simulink model "building_PHPP_carnot83"  (R2023b)
settings: Solver=ode23s  StartTime=-building.preruntime+8760*3600  StopTime=building.runtime+8760*3600  EnableMultiTasking=on
StartFcn:
  | tic
StopFcn:
  | toc
values from neighbouring files (symbols this model uses):
  building = obj    [BUILDING.m]    (also in create_building_automatic.m = building.save(); ini_building_automatic.m = building.add_variant_hvac(building.variant_hvac, hvac); load_building_automatic.m = building.save())
  cp = str2num(value)    [CONSTRUCTION.m]
  p = [timevec_weather weather(:,12)]    [BOUNDARY.m]    (also in WEATHER.m = 0; init_carnotUIBK.m = cell2mat(carnotUIBKpaths(i,2)))
  rho = str2num(value)    [CONSTRUCTION.m]    (also in theta_ground_v1.m = 2000)
undefined symbols (not defined in the file or in its folder): Dreifach, get_building, Qdot_C, Qdot_C_energy, Qdot_H, Qdot_H_energy, Qdot_I_electricity, Qdot_I_electricity_energy, Qdot_I_light, Qdot_I_light_energy, Qdot_I_person, Qdot_I_person_energy, Qdot_S, Qdot_S_energy, Qdot_T_ground, Qdot_T_ground_energy, Qdot_T_neighbour, Qdot_T_neighbour_energy, Qdot_T_opaque, Qdot_T_opaque_energy, Qdot_T_window, Qdot_T_window_energy, Qdot_V_infiltration, Qdot_V_infiltration_energy, Qdot_V_mech, Qdot_V_mech_energy, Qdot_V_window, Qdot_V_window_energy, Tc, Tr, Ts, Wärmeschutzglas, x_CO2, x_H2O, x_VOC
libraries: carnotUIBK x2418, carnot x1
(part 1 of 32)
settings Model: SimulationMode=accelerator  Creator=c8461199  LastModifiedBy=c8461246
settings SolverCC: AlgebraicLoopSolver=TrustRegion
settings DataIOCC: SaveOutput=off  SignalLogging=off  DSMLogging=off  VisualizeSimOutput=off  SaveTime=off  ReturnWorkspaceOutputs=off
settings OptimizationCC: LifeSpan=inf  SimCompilerOptimization=on
settings DebuggingCC: MaxConsecutiveZCsMsg=warning  UnconnectedInputMsg=warning  UnconnectedOutputMsg=warning  UnconnectedLineMsg=warning  AllowSymbolicDim=off  SFUnexpectedBacktrackingDiag=warning  SFNoUnconditionalDefaultTransitionDiag=warning  SFExecutionAtInitializationDiag=none  ArithmeticOperatorsInVariantConditions=warning
settings ModelReferenceCC: EnableRefExpFcnMdlSchedulingChecks=on  EnableParallelModelReferenceBuilds=on  ParallelModelReferenceMATLABWorkerInit=Copy Base Workspace  PropagateSignalLabelsOutOfModel=off
settings SFSimCC: SimUserSources=carlib.c  SimUseLocalCustomCode=off  CustomCodeUndefinedFunction=UseInterfaceOnly
settings RTWCC: RTWUseLocalCustomCode=off  BuildConfiguration=Faster Runs
settings CodeAppCC: StateflowObjectComments=on
settings GRTTargetCC: TargetLangStandard=C89/C90 (ANSI)
settings ConfigComp: CovMetricSettings=dw  CovSaveCumulativeToWorkspaceVar=on  CovSaveSingleToWorkspaceVar=on  CovExternalEMLEnable=off

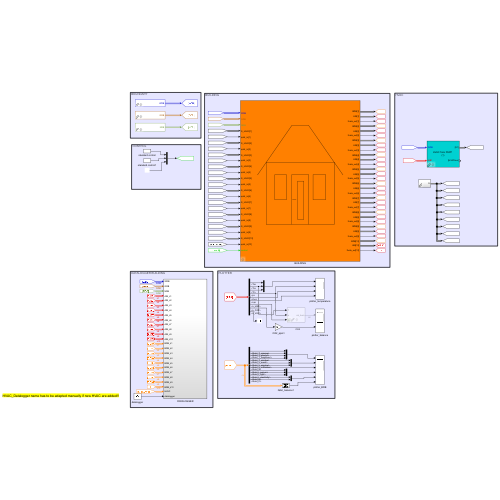
[thumbnail: Simulink's stored preview of the top-level diagram]
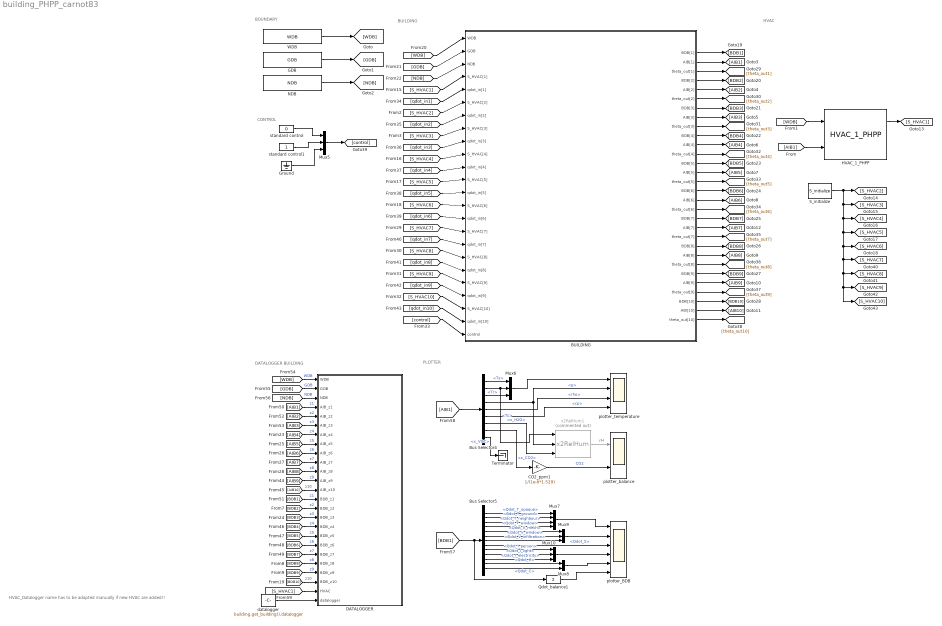
== system building_PHPP_carnot83 ==
  note: HVAC_Datalogger name has to be adapted manually if new HVAC are added!!
  note: PLOTTER
  note: CONTROL
  note: DATALOGGER BUILDING
  note: HVAC
  note: BUILDING
  note: BOUNDARY
  BUILDING : Subsystem  mask{building=get_building(building)}
      mask prompts: building "BUILDING object"
      mask init:
      | b = building;
      mask Display:
      | plot(-20,-30,120,100,[10,10,90,90,10],[0,50,50,0,0],...
      |     [100,60,40,0],[40,80,80,40],[20,34,34,20,20],[40,40,20,20,40],...
      |     [60,60,40,40],[0,40,40,0],[65,80,80,65,65],[40,40,20,20,40],...
      |     [47,54,54,47,47],[35,35,4,4,35],[45,41],[20,20])
  Bus Selector4 : BusSelector  OutputSignals=Ts,Tc,Tr,p,rho,cp,x_H2O,x_CO2,x_VOC
  Bus Selector5 : BusSelector  OutputSignals=Qdot_T_opaque,Qdot_T_ground,Qdot_T_neighbour,Qdot_T_window,Qdot_V_mech,Qdot_V_window,Qdot_V_infiltration,Qdot_S,Qdot_I_person,Qdot_I_light,Qdot_I_electricity,Qdot_H,Qdot_C
  CO2_ppm1 : Gain  Gain=1/(1e-6*1.529)
  DATALOGGER : Subsystem
  GDB : carnotUIBK/boundary/GDB  building=get_building(building)
  Ground : Ground
  HVAC_1_PHPP : carnotUIBK/HVAC/HVAC_1_PHPP  building=get_building(building)  system=1
  Mux10 : Mux  Inputs=3
  Mux5 : Mux  Inputs=[1 1 18]
  Mux6 : Mux  Inputs=3
  Mux7 : Mux
  Mux8 : Mux  Inputs=2
  Mux9 : Mux  Inputs=3
  NDB : carnotUIBK/boundary/NDB  building=get_building(building)
  Qdot_balance1 : Sum  Inputs=1
  S_initialize : carnotUIBK/general/S_initialize  SystemSampleTime=-1  VariantActivationTime=update diagram  AllowFlexibleInterface=on  Latency=0  AutoFrameSizeCalculation=off
  Terminator : Terminator
  WDB : carnotUIBK/boundary/WDB  building=get_building(building)
  datalogger : Constant  Value=building.get_building().datalogger
  plotter_BDB : Scope  NumInputPorts=6
  plotter_balance : Scope  NumInputPorts=2
  plotter_temperature : Scope  NumInputPorts=4
  standard control : Constant  Value=0
  standard control1 : Constant
  x2RelHum1 : carnot/Basic/Material_Properties/x2RelHum  Commented=on
      settings: SourceProductName=Carnot
  wires:
  WDB/1 -> [WDB]
  GDB/1 -> [GDB]
  NDB/1 -> [NDB]
  [WDB] -> BUILDING/1(WDB)
  [GDB] -> BUILDING/2(GDB)
  [NDB] -> BUILDING/3(NDB)
  BUILDING/2(AIB[1]) -> [AIB1]
  BUILDING/5(AIB[2]) -> [AIB2]
  BUILDING/8(AIB[3]) -> [AIB3]
  BUILDING/11(AIB[4]) -> [AIB4]
  BUILDING/14(AIB[5]) -> [AIB5]
  BUILDING/17(AIB[6]) -> [AIB6]
  BUILDING/29(AIB[10]) -> [AIB10]
  BUILDING/26(AIB[9]) -> [AIB9]
  BUILDING/23(AIB[8]) -> [AIB8]
  BUILDING/20(AIB[7]) -> [AIB7]
  [S_HVAC5] -> BUILDING/12(S_HVAC[5])
  [S_HVAC4] -> BUILDING/10(S_HVAC[4])
  [AIB1] -> HVAC_1_PHPP/2
  [S_HVAC1] -> BUILDING/4(S_HVAC[1])
  [S_HVAC2] -> BUILDING/6(S_HVAC[2])
  [S_HVAC3] -> BUILDING/8(S_HVAC[3])
  [S_HVAC6] -> BUILDING/14(S_HVAC[6])
  HVAC_1_PHPP/1 -> [S_HVAC1]
  [S_HVAC10] -> BUILDING/22(S_HVAC[10])
  [S_HVAC9] -> BUILDING/20(S_HVAC[9])
  [S_HVAC8] -> BUILDING/18(S_HVAC[8])
  [S_HVAC7] -> BUILDING/16(S_HVAC[7])
  [control] -> BUILDING/24(control)
  BUILDING/1(BDB[1]) -> [BDB1]
  BUILDING/28(BDB[10]) -> [BDB10]
  BUILDING/4(BDB[2]) -> [BDB2]
  BUILDING/7(BDB[3]) -> [BDB3]
  BUILDING/10(BDB[4]) -> [BDB4]
  BUILDING/13(BDB[5]) -> [BDB5]
  BUILDING/16(BDB[6]) -> [BDB6]
  BUILDING/19(BDB[7]) -> [BDB7]
  BUILDING/22(BDB[8]) -> [BDB8]
  BUILDING/25(BDB[9]) -> [BDB9]
  [qdot_in1] -> BUILDING/5(qdot_in[1])
  [qdot_in9] -> BUILDING/21(qdot_in[9])
  [qdot_in10] -> BUILDING/23(qdot_in[10])
  [qdot_in8] -> BUILDING/19(qdot_in[8])
  [qdot_in7] -> BUILDING/17(qdot_in[7])
  [qdot_in6] -> BUILDING/15(qdot_in[6])
  [qdot_in4] -> BUILDING/11(qdot_in[4])
  [qdot_in5] -> BUILDING/13(qdot_in[5])
  [qdot_in3] -> BUILDING/9(qdot_in[3])
  [qdot_in2] -> BUILDING/7(qdot_in[2])
  BUILDING/3(theta_out[1]) -> [theta_out1]
  BUILDING/30(theta_out[10]) -> [theta_out10]
  BUILDING/27(theta_out[9]) -> [theta_out9]
  BUILDING/24(theta_out[8]) -> [theta_out8]
  BUILDING/21(theta_out[7]) -> [theta_out7]
  BUILDING/18(theta_out[6]) -> [theta_out6]
  BUILDING/15(theta_out[5]) -> [theta_out5]
  BUILDING/12(theta_out[4]) -> [theta_out4]
  BUILDING/9(theta_out[3]) -> [theta_out3]
  BUILDING/6(theta_out[2]) -> [theta_out2]
  datalogger/1 -> DATALOGGER/25(datalogger)
  standard control/1 -> Mux5/1
  Mux5/1 -> [control]
  Ground/1 -> Mux5/3
  [AIB1] -> DATALOGGER/4(AIB_z1)  "z1"
  [WDB] -> DATALOGGER/1(WDB)  "WDB"
  [GDB] -> DATALOGGER/2(GDB)  "GDB"
  [NDB] -> DATALOGGER/3(NDB)  "NDB"
  [AIB2] -> DATALOGGER/5(AIB_z2)  "z2"
  [AIB3] -> DATALOGGER/6(AIB_z3)  "z3"
  [AIB4] -> DATALOGGER/7(AIB_z4)  "z4"
  [AIB5] -> DATALOGGER/8(AIB_z5)  "z5"
  [AIB6] -> DATALOGGER/9(AIB_z6)  "z6"
  [AIB7] -> DATALOGGER/10(AIB_z7)  "z7"
  [AIB8] -> DATALOGGER/11(AIB_z8)  "z8"
  [AIB9] -> DATALOGGER/12(AIB_z9)  "z9"
  [AIB10] -> DATALOGGER/13(AIB_z10)  "z10"
  [BDB1] -> DATALOGGER/14(BDB_z1)  "z1"
  [BDB2] -> DATALOGGER/15(BDB_z2)  "z2"
  [BDB3] -> DATALOGGER/16(BDB_z3)  "z3"
  [BDB4] -> DATALOGGER/17(BDB_z4)  "z4"
  [BDB5] -> DATALOGGER/18(BDB_z5)  "z5"
  [BDB6] -> DATALOGGER/19(BDB_z6)  "z6"
  [BDB7] -> DATALOGGER/20(BDB_z7)  "z7"
  [BDB8] -> DATALOGGER/21(BDB_z8)  "z8"
  [BDB9] -> DATALOGGER/22(BDB_z9)  "z9"
  [BDB10] -> DATALOGGER/23(BDB_z10)  "z10"
  Bus Selector4/4 -> x2RelHum1/2, plotter_temperature/2  "<p>"
  Bus Selector4/1 -> Mux6/1  "<Ts>"
  Bus Selector4/2 -> x2RelHum1/1, Mux6/2  "<Tc>"
  Bus Selector4/3 -> Mux6/3  "<Tr>"
  Mux6/1 -> plotter_temperature/1
  Bus Selector4/5 -> plotter_temperature/3  "<rho>"
  Bus Selector4/6 -> plotter_temperature/4  "<cp>"
  Bus Selector4/8 -> CO2_ppm1/1  "<x_CO2>"
  CO2_ppm1/1 -> plotter_balance/2  "CO2"
  Bus Selector4/7 -> x2RelHum1/3  "<x_H2O>"
  x2RelHum1/1 -> plotter_balance/1  "rH"
  Bus Selector5/6 -> Mux9/2  "<Qdot_V_window>"
  Bus Selector5/5 -> Mux9/1  "<Qdot_V_mech>"
  Bus Selector5/4 -> Mux7/4  "<Qdot_T_window>"
  Bus Selector5/3 -> Mux7/3  "<Qdot_T_neighbour>"
  Bus Selector5/2 -> Mux7/2  "<Qdot_T_ground>"
  Bus Selector5/1 -> Mux7/1  "<Qdot_T_opaque>"
  Bus Selector5/7 -> Mux9/3  "<Qdot_V_infiltration>"
  Bus Selector5/8 -> plotter_BDB/3  "<Qdot_S>"
  Bus Selector5/9 -> Mux10/1  "<Qdot_I_person>"
  Bus Selector5/10 -> Mux10/2  "<Qdot_I_light>"
  Bus Selector5/11 -> Mux10/3  "<Qdot_I_electricity>"
  Mux7/1 -> plotter_BDB/1
  [BDB1] -> Qdot_balance1/1, Bus Selector5/1
  Mux9/1 -> plotter_BDB/2
  Mux10/1 -> plotter_BDB/4
  Bus Selector5/12 -> Mux8/1  "<Qdot_H>"
  Bus Selector5/13 -> Mux8/2  "<Qdot_C>"
  Mux8/1 -> plotter_BDB/5
  Qdot_balance1/1 -> plotter_BDB/6
  [AIB1] -> Bus Selector4/1
  [S_HVAC1] -> DATALOGGER/24(HVAC)
  standard control1/1 -> Mux5/2
  [WDB] -> HVAC_1_PHPP/1
  Bus Selector4/9 -> Terminator/1  "<x_VOC>"
  S_initialize/1 -> [S_HVAC2], [S_HVAC3], [S_HVAC4], [S_HVAC6], [S_HVAC7], [S_HVAC8], [S_HVAC9], [S_HVAC10], [S_HVAC5]

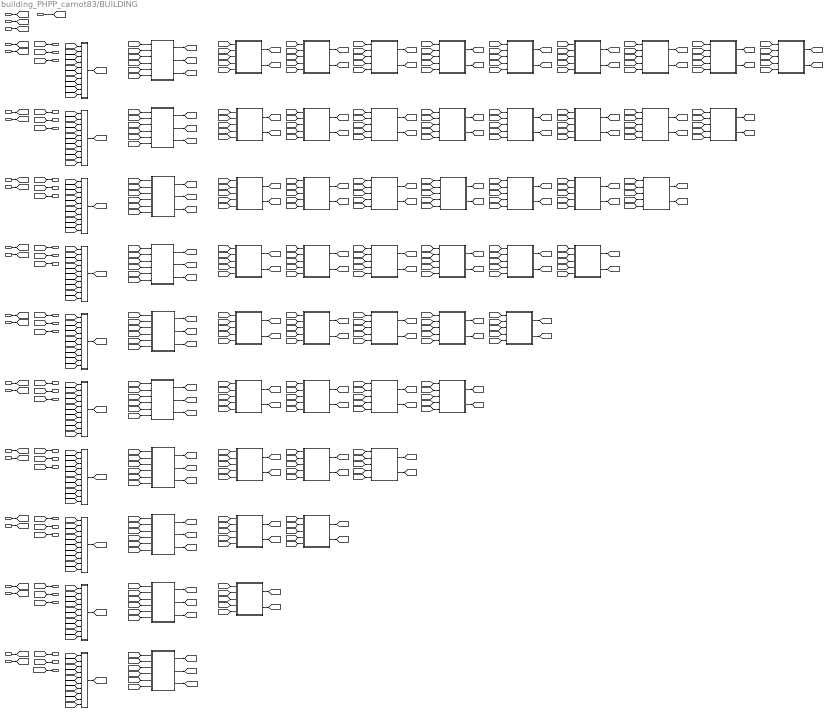
== system building_PHPP_carnot83/BUILDING ==
  note: INTERSECTION 1_2
  note: ZONE 1
  note: ZONE 1 - SUM UP S
  note: ZONE 6 - INPUT AND OUTPUT
  note: ZONE 5 - INPUT AND OUTPUT
  note: ZONE 4 - INPUT AND OUTPUT
  note: ZONE 3 - INPUT AND OUTPUT
  note: ZONE 2 - INPUT AND OUTPUT
  note: ZONE 1 - INPUT AND OUTPUT
  note: BUS BOUNDARY
  note: ZONE 2 - SUM UP S
  note: ZONE 3 - SUM UP S
  note: ZONE 4 - SUM UP S
  note: ZONE 5 - SUM UP S
  note: ZONE 6 - SUM UP S
  note: ZONE 7 - INPUT AND OUTPUT
  note: ZONE 7 - SUM UP S
  note: ZONE 8 - INPUT AND OUTPUT
  note: ZONE 8 - SUM UP S
  note: ZONE 9 - INPUT AND OUTPUT
  note: ZONE 9 - SUM UP S
  note: ZONE 10 - INPUT AND OUTPUT
  note: ZONE 10 - SUM UP S
  note: ZONE 2
  note: ZONE 3
  note: ZONE 4
  note: ZONE 5
  note: ZONE6
  note: ZONE 7
  note: ZONE 8
  note: ZONE 9
  note: ZONE 10
  note: CONTROL
  note: INTERSECTION 1_10
  note: INTERSECTION 1_3
  note: INTERSECTION 1_4
  note: INTERSECTION 1_5
  note: INTERSECTION 1_6
  note: INTERSECTION 1_7
  note: INTERSECTION 1_8
  note: INTERSECTION 1_9
  note: INTERSECTION 2_3
  note: INTERSECTION 2_9
  note: INTERSECTION 2_10
  note: INTERSECTION 2_4
  note: INTERSECTION 2_5
  note: INTERSECTION 2_6
  note: INTERSECTION 2_7
  note: INTERSECTION 2_8
  note: INTERSECTION 3_4
  note: INTERSECTION 3_5
  note: INTERSECTION 3_6
  note: INTERSECTION 3_7
  note: INTERSECTION 3_8
  note: INTERSECTION 3_9
  note: INTERSECTION 3_10
  note: INTERSECTION 4_5
  note: INTERSECTION 4_6
  note: INTERSECTION 4_7
  note: INTERSECTION 4_8
  note: INTERSECTION 4_9
  note: INTERSECTION 4_10
  note: INTERSECTION 5_6
  note: INTERSECTION 5_7
  note: INTERSECTION 5_8
  note: INTERSECTION 5_9
  note: INTERSECTION 5_10
  note: INTERSECTION 6_7
  note: INTERSECTION 6_8
  note: INTERSECTION 6_9
  note: INTERSECTION 6_10
  note: INTERSECTION 7_8
  note: INTERSECTION 7_9
  note: INTERSECTION 7_10
  note: INTERSECTION 8_9
  note: INTERSECTION 8_10
  note: INTERSECTION 9_10
  WDB : Inport
  GDB : Inport  Port=2
  NDB : Inport  Port=3
  S_HVAC[1] : Inport  Port=4
  qdot_in[1] : Inport  Port=5
  S_HVAC[2] : Inport  Port=6
  qdot_in[2] : Inport  Port=7
  S_HVAC[3] : Inport  Port=8
  qdot_in[3] : Inport  Port=9
  S_HVAC[4] : Inport  Port=10
  qdot_in[4] : Inport  Port=11
  S_HVAC[5] : Inport  Port=12
  qdot_in[5] : Inport  Port=13
  S_HVAC[6] : Inport  Port=14
  qdot_in[6] : Inport  Port=15
  S_HVAC[7] : Inport  Port=16
  qdot_in[7] : Inport  Port=17
  S_HVAC[8] : Inport  Port=18
  qdot_in[8] : Inport  Port=19
  S_HVAC[9] : Inport  Port=20
  qdot_in[9] : Inport  Port=21
  S_HVAC[10] : Inport  Port=22
  qdot_in[10] : Inport  Port=23
  control : Inport  Port=24
  INTERSECTION_1_10 : Subsystem  VariantControl=Variant1  mask{intersection=b.thermalzone.intersection{1,10}}
      mask prompts: intersection "INTERSECTION object"
      mask init:
      | i = intersection;
      | z = intersection;
      mask Display: fprintf('%s',intersection.name)
  INTERSECTION_1_2 : Subsystem  VariantControl=Variant1  mask{intersection=b.thermalzone.intersection{1,2}}
      mask prompts: intersection "INTERSECTION object"
      mask init:
      | i = intersection;
      | z = intersection;
      mask Display: fprintf('%s',intersection.name)
  INTERSECTION_1_3 : Subsystem  VariantControl=Variant1  mask{intersection=b.thermalzone.intersection{1,3}}
      mask prompts: intersection "INTERSECTION object"
      mask init:
      | i = intersection;
      | z = intersection;
      mask Display: fprintf('%s',intersection.name)
  INTERSECTION_1_4 : Subsystem  VariantControl=Variant1  mask{intersection=b.thermalzone.intersection{1,4}}
      mask prompts: intersection "INTERSECTION object"
      mask init:
      | i = intersection;
      | z = intersection;
      mask Display: fprintf('%s',intersection.name)
  INTERSECTION_1_5 : Subsystem  VariantControl=Variant1  mask{intersection=b.thermalzone.intersection{1,5}}
      mask prompts: intersection "INTERSECTION object"
      mask init:
      | i = intersection;
      | z = intersection;
      mask Display: fprintf('%s',intersection.name)
  INTERSECTION_1_6 : Subsystem  VariantControl=Variant1  mask{intersection=b.thermalzone.intersection{1,6}}
      mask prompts: intersection "INTERSECTION object"
      mask init:
      | i = intersection;
      | z = intersection;
      mask Display: fprintf('%s',intersection.name)
  INTERSECTION_1_7 : Subsystem  VariantControl=Variant1  mask{intersection=b.thermalzone.intersection{1,7}}
      mask prompts: intersection "INTERSECTION object"
      mask init:
      | i = intersection;
      | z = intersection;
      mask Display: fprintf('%s',intersection.name)
  INTERSECTION_1_8 : Subsystem  VariantControl=Variant1  mask{intersection=b.thermalzone.intersection{1,8}}
      mask prompts: intersection "INTERSECTION object"
      mask init:
      | i = intersection;
      | z = intersection;
      mask Display: fprintf('%s',intersection.name)
  INTERSECTION_1_9 : Subsystem  VariantControl=Variant1  mask{intersection=b.thermalzone.intersection{1,9}}
      mask prompts: intersection "INTERSECTION object"
      mask init:
      | i = intersection;
      | z = intersection;
      mask Display: fprintf('%s',intersection.name)
  INTERSECTION_2_10 : Subsystem  VariantControl=Variant1  mask{intersection=b.thermalzone.intersection{2,10}}
      mask prompts: intersection "INTERSECTION object"
      mask init:
      | i = intersection;
      | z = intersection;
      mask Display: fprintf('%s',intersection.name)
  INTERSECTION_2_3 : Subsystem  VariantControl=Variant1  mask{intersection=b.thermalzone.intersection{2,3}}
      mask prompts: intersection "INTERSECTION object"
      mask init:
      | i = intersection;
      | z = intersection;
      mask Display: fprintf('%s',intersection.name)
  INTERSECTION_2_4 : Subsystem  VariantControl=Variant1  mask{intersection=b.thermalzone.intersection{2,4}}
      mask prompts: intersection "INTERSECTION object"
      mask init:
      | i = intersection;
      | z = intersection;
      mask Display: fprintf('%s',intersection.name)
  INTERSECTION_2_5 : Subsystem  VariantControl=Variant1  mask{intersection=b.thermalzone.intersection{2,5}}
      mask prompts: intersection "INTERSECTION object"
      mask init:
      | i = intersection;
      | z = intersection;
      mask Display: fprintf('%s',intersection.name)
  INTERSECTION_2_6 : Subsystem  VariantControl=Variant1  mask{intersection=b.thermalzone.intersection{2,6}}
      mask prompts: intersection "INTERSECTION object"
      mask init:
      | i = intersection;
      | z = intersection;
      mask Display: fprintf('%s',intersection.name)
  INTERSECTION_2_7 : Subsystem  VariantControl=Variant1  mask{intersection=b.thermalzone.intersection{2,7}}
      mask prompts: intersection "INTERSECTION object"
      mask init:
      | i = intersection;
      | z = intersection;
      mask Display: fprintf('%s',intersection.name)
  INTERSECTION_2_8 : Subsystem  VariantControl=Variant1  mask{intersection=b.thermalzone.intersection{2,8}}
      mask prompts: intersection "INTERSECTION object"
      mask init:
      | i = intersection;
      | z = intersection;
      mask Display: fprintf('%s',intersection.name)
  INTERSECTION_2_9 : Subsystem  VariantControl=Variant1  mask{intersection=b.thermalzone.intersection{2,9}}
      mask prompts: intersection "INTERSECTION object"
      mask init:
      | i = intersection;
      | z = intersection;
      mask Display: fprintf('%s',intersection.name)
  INTERSECTION_3_10 : Subsystem  VariantControl=Variant1  mask{intersection=b.thermalzone.intersection{3,10}}
      mask prompts: intersection "INTERSECTION object"
      mask init:
      | i = intersection;
      | z = intersection;
      mask Display: fprintf('%s',intersection.name)
  INTERSECTION_3_4 : Subsystem  VariantControl=Variant1  mask{intersection=b.thermalzone.intersection{3,4}}
      mask prompts: intersection "INTERSECTION object"
      mask init:
      | i = intersection;
      | z = intersection;
      mask Display: fprintf('%s',intersection.name)
  INTERSECTION_3_5 : Subsystem  VariantControl=Variant1  mask{intersection=b.thermalzone.intersection{3,5}}
      mask prompts: intersection "INTERSECTION object"
      mask init:
      | i = intersection;
      | z = intersection;
      mask Display: fprintf('%s',intersection.name)
  INTERSECTION_3_6 : Subsystem  VariantControl=Variant1  mask{intersection=b.thermalzone.intersection{3,6}}
      mask prompts: intersection "INTERSECTION object"
      mask init:
      | i = intersection;
      | z = intersection;
      mask Display: fprintf('%s',intersection.name)
  INTERSECTION_3_7 : Subsystem  VariantControl=Variant1  mask{intersection=b.thermalzone.intersection{3,7}}
      mask prompts: intersection "INTERSECTION object"
      mask init:
      | i = intersection;
      | z = intersection;
      mask Display: fprintf('%s',intersection.name)
  INTERSECTION_3_8 : Subsystem  VariantControl=Variant1  mask{intersection=b.thermalzone.intersection{3,8}}
      mask prompts: intersection "INTERSECTION object"
      mask init:
      | i = intersection;
      | z = intersection;
      mask Display: fprintf('%s',intersection.name)
  INTERSECTION_3_9 : Subsystem  VariantControl=Variant1  mask{intersection=b.thermalzone.intersection{3,9}}
      mask prompts: intersection "INTERSECTION object"
      mask init:
      | i = intersection;
      | z = intersection;
      mask Display: fprintf('%s',intersection.name)
  INTERSECTION_4_10 : Subsystem  VariantControl=Variant1  mask{intersection=b.thermalzone.intersection{4,10}}
      mask prompts: intersection "INTERSECTION object"
      mask init:
      | i = intersection;
      | z = intersection;
      mask Display: fprintf('%s',intersection.name)
  INTERSECTION_4_5 : Subsystem  VariantControl=Variant1  mask{intersection=b.thermalzone.intersection{4,5}}
      mask prompts: intersection "INTERSECTION object"
      mask init:
      | i = intersection;
      | z = intersection;
      mask Display: fprintf('%s',intersection.name)
  INTERSECTION_4_6 : Subsystem  VariantControl=Variant1  mask{intersection=b.thermalzone.intersection{4,6}}
      mask prompts: intersection "INTERSECTION object"
      mask init:
      | i = intersection;
      | z = intersection;
      mask Display: fprintf('%s',intersection.name)
  INTERSECTION_4_7 : Subsystem  VariantControl=Variant1  mask{intersection=b.thermalzone.intersection{4,7}}
      mask prompts: intersection "INTERSECTION object"
      mask init:
      | i = intersection;
      | z = intersection;
      mask Display: fprintf('%s',intersection.name)
  INTERSECTION_4_8 : Subsystem  VariantControl=Variant1  mask{intersection=b.thermalzone.intersection{4,8}}
      mask prompts: intersection "INTERSECTION object"
      mask init:
      | i = intersection;
      | z = intersection;
      mask Display: fprintf('%s',intersection.name)
  INTERSECTION_4_9 : Subsystem  VariantControl=Variant1  mask{intersection=b.thermalzone.intersection{4,9}}
      mask prompts: intersection "INTERSECTION object"
      mask init:
      | i = intersection;
      | z = intersection;
      mask Display: fprintf('%s',intersection.name)
  INTERSECTION_5_10 : Subsystem  VariantControl=Variant1  mask{intersection=b.thermalzone.intersection{5,10}}
      mask prompts: intersection "INTERSECTION object"
      mask init:
      | i = intersection;
      | z = intersection;
      mask Display: fprintf('%s',intersection.name)
  INTERSECTION_5_6 : Subsystem  VariantControl=Variant1  mask{intersection=b.thermalzone.intersection{5,6}}
      mask prompts: intersection "INTERSECTION object"
      mask init:
      | i = intersection;
      | z = intersection;
      mask Display: fprintf('%s',intersection.name)
  INTERSECTION_5_7 : Subsystem  VariantControl=Variant1  mask{intersection=b.thermalzone.intersection{5,7}}
      mask prompts: intersection "INTERSECTION object"
      mask init:
      | i = intersection;
      | z = intersection;
      mask Display: fprintf('%s',intersection.name)
  INTERSECTION_5_8 : Subsystem  VariantControl=Variant1  mask{intersection=b.thermalzone.intersection{5,8}}
      mask prompts: intersection "INTERSECTION object"
      mask init:
      | i = intersection;
      | z = intersection;
      mask Display: fprintf('%s',intersection.name)
  INTERSECTION_5_9 : Subsystem  VariantControl=Variant1  mask{intersection=b.thermalzone.intersection{5,9}}
      mask prompts: intersection "INTERSECTION object"
      mask init:
      | i = intersection;
      | z = intersection;
      mask Display: fprintf('%s',intersection.name)
  INTERSECTION_6_10 : Subsystem  VariantControl=Variant1  mask{intersection=b.thermalzone.intersection{6,10}}
      mask prompts: intersection "INTERSECTION object"
      mask init:
      | i = intersection;
      | z = intersection;
      mask Display: fprintf('%s',intersection.name)
  INTERSECTION_6_7 : Subsystem  VariantControl=Variant1  mask{intersection=b.thermalzone.intersection{6,7}}
      mask prompts: intersection "INTERSECTION object"
      mask init:
      | i = intersection;
      | z = intersection;
      mask Display: fprintf('%s',intersection.name)
  INTERSECTION_6_8 : Subsystem  VariantControl=Variant1  mask{intersection=b.thermalzone.intersection{6,8}}
      mask prompts: intersection "INTERSECTION object"
      mask init:
      | i = intersection;
      | z = intersection;
      mask Display: fprintf('%s',intersection.name)
  INTERSECTION_6_9 : Subsystem  VariantControl=Variant1  mask{intersection=b.thermalzone.intersection{6,9}}
      mask prompts: intersection "INTERSECTION object"
      mask init:
      | i = intersection;
      | z = intersection;
      mask Display: fprintf('%s',intersection.name)
  INTERSECTION_7_10 : Subsystem  VariantControl=Variant1  mask{intersection=b.thermalzone.intersection{7,10}}
      mask prompts: intersection "INTERSECTION object"
      mask init:
      | i = intersection;
      | z = intersection;
      mask Display: fprintf('%s',intersection.name)
  INTERSECTION_7_8 : Subsystem  VariantControl=Variant1  mask{intersection=b.thermalzone.intersection{7,8}}
      mask prompts: intersection "INTERSECTION object"
      mask init:
      | i = intersection;
      | z = intersection;
      mask Display: fprintf('%s',intersection.name)
  INTERSECTION_7_9 : Subsystem  VariantControl=Variant1  mask{intersection=b.thermalzone.intersection{7,9}}
      mask prompts: intersection "INTERSECTION object"
      mask init:
      | i = intersection;
      | z = intersection;
      mask Display: fprintf('%s',intersection.name)
  INTERSECTION_8_10 : Subsystem  VariantControl=Variant1  mask{intersection=b.thermalzone.intersection{8,10}}
      mask prompts: intersection "INTERSECTION object"
      mask init:
      | i = intersection;
      | z = intersection;
      mask Display: fprintf('%s',intersection.name)
  INTERSECTION_8_9 : Subsystem  VariantControl=Variant1  mask{intersection=b.thermalzone.intersection{8,9}}
      mask prompts: intersection "INTERSECTION object"
      mask init:
      | i = intersection;
      | z = intersection;
      mask Display: fprintf('%s',intersection.name)
  INTERSECTION_9_10 : Subsystem  VariantControl=Variant1  mask{intersection=b.thermalzone.intersection{9,10}}
      mask prompts: intersection "INTERSECTION object"
      mask init:
      | i = intersection;
      | z = intersection;
      mask Display: fprintf('%s',intersection.name)
  Subsystem : Subsystem
  Subsystem1 : Subsystem
  Subsystem2 : Subsystem
  Subsystem3 : Subsystem
  Subsystem4 : Subsystem
  Subsystem5 : Subsystem
  Subsystem6 : Subsystem
  Subsystem7 : Subsystem
  Subsystem8 : Subsystem
  Subsystem9 : Subsystem
  ZONE_1 : Subsystem  mask{zone=b.thermalzone.zone(1)}
      mask prompts: zone "ZONE object"
      mask init:
      | z = zone;
      mask Display: fprintf('%s',zone.name)
  ZONE_10 : Subsystem  mask{zone=b.thermalzone.zone(10)}
      mask prompts: zone "ZONE object"
      mask init:
      | z = zone;
      mask Display: fprintf('%s',zone.name)
  ZONE_2 : Subsystem  mask{zone=b.thermalzone.zone(2)}
      mask prompts: zone "ZONE object"
      mask init:
      | z = zone;
      mask Display: fprintf('%s',zone.name)
  ZONE_3 : Subsystem  mask{zone=b.thermalzone.zone(3)}
      mask prompts: zone "ZONE object"
      mask init:
      | z = zone;
      mask Display: fprintf('%s',zone.name)
  ZONE_4 : Subsystem  mask{zone=b.thermalzone.zone(4)}
      mask prompts: zone "ZONE object"
      mask init:
      | z = zone;
      mask Display: fprintf('%s',zone.name)
  ZONE_5 : Subsystem  mask{zone=b.thermalzone.zone(5)}
      mask prompts: zone "ZONE object"
      mask init:
      | z = zone;
      mask Display: fprintf('%s',zone.name)
  ZONE_6 : Subsystem  mask{zone=b.thermalzone.zone(6)}
      mask prompts: zone "ZONE object"
      mask init:
      | z = zone;
      mask Display: fprintf('%s',zone.name)
  ZONE_7 : Subsystem  mask{zone=b.thermalzone.zone(7)}
      mask prompts: zone "ZONE object"
      mask init:
      | z = zone;
      mask Display: fprintf('%s',zone.name)
  ZONE_8 : Subsystem  mask{zone=b.thermalzone.zone(8)}
      mask prompts: zone "ZONE object"
      mask init:
      | z = zone;
      mask Display: fprintf('%s',zone.name)
  ZONE_9 : Subsystem  mask{zone=b.thermalzone.zone(9)}
      mask prompts: zone "ZONE object"
      mask init:
      | z = zone;
      mask Display: fprintf('%s',zone.name)
  BDB[1] : Outport  VectorParamsAs1DForOutWhenUnconnected=off
  AIB[1] : Outport  Port=2  VectorParamsAs1DForOutWhenUnconnected=off
  theta_out[1] : Outport  Port=3  VectorParamsAs1DForOutWhenUnconnected=off
  BDB[2] : Outport  Port=4  VectorParamsAs1DForOutWhenUnconnected=off
  AIB[2] : Outport  Port=5  VectorParamsAs1DForOutWhenUnconnected=off
  theta_out[2] : Outport  Port=6  VectorParamsAs1DForOutWhenUnconnected=off
  BDB[3] : Outport  Port=7  VectorParamsAs1DForOutWhenUnconnected=off
  AIB[3] : Outport  Port=8  VectorParamsAs1DForOutWhenUnconnected=off
  theta_out[3] : Outport  Port=9  VectorParamsAs1DForOutWhenUnconnected=off
  BDB[4] : Outport  Port=10  VectorParamsAs1DForOutWhenUnconnected=off
  AIB[4] : Outport  Port=11  VectorParamsAs1DForOutWhenUnconnected=off
  theta_out[4] : Outport  Port=12  VectorParamsAs1DForOutWhenUnconnected=off
  BDB[5] : Outport  Port=13  VectorParamsAs1DForOutWhenUnconnected=off
  AIB[5] : Outport  Port=14  VectorParamsAs1DForOutWhenUnconnected=off
  theta_out[5] : Outport  Port=15  VectorParamsAs1DForOutWhenUnconnected=off
  BDB[6] : Outport  Port=16  VectorParamsAs1DForOutWhenUnconnected=off
  AIB[6] : Outport  Port=17  VectorParamsAs1DForOutWhenUnconnected=off
  theta_out[6] : Outport  Port=18  VectorParamsAs1DForOutWhenUnconnected=off
  BDB[7] : Outport  Port=19  VectorParamsAs1DForOutWhenUnconnected=off
  AIB[7] : Outport  Port=20  VectorParamsAs1DForOutWhenUnconnected=off
  theta_out[7] : Outport  Port=21  VectorParamsAs1DForOutWhenUnconnected=off
  BDB[8] : Outport  Port=22  VectorParamsAs1DForOutWhenUnconnected=off
  AIB[8] : Outport  Port=23  VectorParamsAs1DForOutWhenUnconnected=off
  theta_out[8] : Outport  Port=24  VectorParamsAs1DForOutWhenUnconnected=off
  BDB[9] : Outport  Port=25  VectorParamsAs1DForOutWhenUnconnected=off
  AIB[9] : Outport  Port=26  VectorParamsAs1DForOutWhenUnconnected=off
  theta_out[9] : Outport  Port=27  VectorParamsAs1DForOutWhenUnconnected=off
  BDB[10] : Outport  Port=28  VectorParamsAs1DForOutWhenUnconnected=off
  AIB[10] : Outport  Port=29  VectorParamsAs1DForOutWhenUnconnected=off
  theta_out[10] : Outport  Port=30  VectorParamsAs1DForOutWhenUnconnected=off
  wires:
  WDB/1 -> [WDB]
  GDB/1 -> [GDB]
  NDB/1 -> [NDB]
  S_HVAC[1]/1 -> [S_HVAC_1]
  qdot_in[1]/1 -> [qdot_in_1]
  [BDB_1] -> BDB[1]/1
  [AIB_1] -> AIB[1]/1
  [theta_out_1z] -> theta_out[1]/1
  S_HVAC[2]/1 -> [S_HVAC_2]
  qdot_in[2]/1 -> [qdot_in_2]
  qdot_in[3]/1 -> [qdot_in_3]
  S_HVAC[3]/1 -> [S_HVAC_3]
  S_HVAC[4]/1 -> [S_HVAC_4]
  qdot_in[4]/1 -> [qdot_in_4]
  S_HVAC[5]/1 -> [S_HVAC_5]
  qdot_in[5]/1 -> [qdot_in_5]
  qdot_in[6]/1 -> [qdot_in_6]
  S_HVAC[6]/1 -> [S_HVAC_6]
  [BDB_2] -> BDB[2]/1
  [AIB_2] -> AIB[2]/1
  [theta_out_2z] -> theta_out[2]/1
  [BDB_3] -> BDB[3]/1
  [AIB_3] -> AIB[3]/1
  [theta_out_3z] -> theta_out[3]/1
  [BDB_4] -> BDB[4]/1
  [AIB_4] -> AIB[4]/1
  [theta_out_4z] -> theta_out[4]/1
  [BDB_5] -> BDB[5]/1
  [AIB_5] -> AIB[5]/1
  [theta_out_5z] -> theta_out[5]/1
  [BDB_6] -> BDB[6]/1
  [AIB_6] -> AIB[6]/1
  [theta_out_6z] -> theta_out[6]/1
  ZONE_1/1(BDB) -> [BDB_1]
  ZONE_1/2(AIB) -> [AIB_1]
  ZONE_1/3(theta_out) -> [theta_out_1z]
  [qdot_in_1] -> ZONE_1/5(Qdot_in)
  [S_in_1] -> ZONE_1/4(S_in)
  [GDB] -> ZONE_1/2(GDB)
  [NDB] -> ZONE_1/3(NDB)
  [S_HVAC_1] -> Subsystem/1(S1)
  [S_I_16] -> Subsystem/6(S6)
  [S_I_12] -> Subsystem/2(S2)
  [S_I_13] -> Subsystem/3(S3)
  [S_I_14] -> Subsystem/4(S4)
  [S_I_15] -> Subsystem/5(S5)
  Subsystem/1(Sout) -> [S_in_1]
  [S_HVAC_2] -> Subsystem1/1(S1)
  Subsystem1/1(Sout) -> [S_in_2]
  Subsystem2/1(Sout) -> [S_in_3]
  Subsystem3/1(Sout) -> [S_in_4]
  Subsystem4/1(Sout) -> [S_in_5]
  Subsystem5/1(Sout) -> [S_in_6]
  [S_I_17] -> Subsystem/7(S7)
  [S_I_18] -> Subsystem/8(S8)
  [S_I_19] -> Subsystem/9(S9)
  [S_I_110] -> Subsystem/10(S10)
  [S_I_27] -> Subsystem1/7(S7)
  [S_I_28] -> Subsystem1/8(S8)
  [S_I_29] -> Subsystem1/9(S9)
  [S_I_210] -> Subsystem1/10(S10)
  [S_I_21] -> Subsystem1/2(S2)
  [S_I_23] -> Subsystem1/3(S3)
  [S_I_26] -> Subsystem1/6(S6)
  [S_I_25] -> Subsystem1/5(S5)
  [S_I_24] -> Subsystem1/4(S4)
  [S_I_37] -> Subsystem2/7(S7)
  [S_I_38] -> Subsystem2/8(S8)
  [S_I_39] -> Subsystem2/9(S9)
  [S_I_310] -> Subsystem2/10(S10)
  [S_HVAC_3] -> Subsystem2/1(S1)
  [S_I_31] -> Subsystem2/2(S2)
  [S_I_32] -> Subsystem2/3(S3)
  [S_I_34] -> Subsystem2/4(S4)
  [S_I_35] -> Subsystem2/5(S5)
  [S_I_36] -> Subsystem2/6(S6)
  [S_I_47] -> Subsystem3/7(S7)
  [S_I_48] -> Subsystem3/8(S8)
  [S_I_49] -> Subsystem3/9(S9)
  [S_I_410] -> Subsystem3/10(S10)
  [S_HVAC_4] -> Subsystem3/1(S1)
  [S_I_41] -> Subsystem3/2(S2)
  [S_I_42] -> Subsystem3/3(S3)
  [S_I_43] -> Subsystem3/4(S4)
  [S_I_45] -> Subsystem3/5(S5)
  [S_I_46] -> Subsystem3/6(S6)
  [S_I_57] -> Subsystem4/7(S7)
  [S_I_58] -> Subsystem4/8(S8)
  [S_I_59] -> Subsystem4/9(S9)
  [S_I_510] -> Subsystem4/10(S10)
  [S_HVAC_5] -> Subsystem4/1(S1)
  [S_I_51] -> Subsystem4/2(S2)
  [S_I_52] -> Subsystem4/3(S3)
  [S_I_53] -> Subsystem4/4(S4)
  [S_I_54] -> Subsystem4/5(S5)
  [S_I_56] -> Subsystem4/6(S6)
  [S_I_67] -> Subsystem5/7(S7)
  [S_I_68] -> Subsystem5/8(S8)
  [S_I_69] -> Subsystem5/9(S9)
  [S_I_610] -> Subsystem5/10(S10)
  [S_HVAC_6] -> Subsystem5/1(S1)
  [S_I_61] -> Subsystem5/2(S2)
  [S_I_62] -> Subsystem5/3(S3)
  [S_I_63] -> Subsystem5/4(S4)
  [S_I_64] -> Subsystem5/5(S5)
  [S_I_65] -> Subsystem5/6(S6)
  qdot_in[7]/1 -> [qdot_in_7]
  S_HVAC[7]/1 -> [S_HVAC_7]
  [BDB_7] -> BDB[7]/1
  [AIB_7] -> AIB[7]/1
  [theta_out_7z] -> theta_out[7]/1
  Subsystem6/1(Sout) -> [S_in_7]
  [S_I_76] -> Subsystem6/7(S7)
  [S_I_78] -> Subsystem6/8(S8)
  [S_I_79] -> Subsystem6/9(S9)
  [S_I_710] -> Subsystem6/10(S10)
  [S_HVAC_7] -> Subsystem6/1(S1)
  [S_I_71] -> Subsystem6/2(S2)
  [S_I_72] -> Subsystem6/3(S3)
  [S_I_73] -> Subsystem6/4(S4)
  [S_I_74] -> Subsystem6/5(S5)
  [S_I_75] -> Subsystem6/6(S6)
  qdot_in[8]/1 -> [qdot_in_8]
  S_HVAC[8]/1 -> [S_HVAC_8]
  [BDB_8] -> BDB[8]/1
  [AIB_8] -> AIB[8]/1
  [theta_out_8z] -> theta_out[8]/1
  Subsystem7/1(Sout) -> [S_in_8]
  [S_I_86] -> Subsystem7/7(S7)
  [S_I_87] -> Subsystem7/8(S8)
  [S_I_89] -> Subsystem7/9(S9)
  [S_I_810] -> Subsystem7/10(S10)
  [S_HVAC_8] -> Subsystem7/1(S1)
  [S_I_81] -> Subsystem7/2(S2)
  [S_I_82] -> Subsystem7/3(S3)
  [S_I_83] -> Subsystem7/4(S4)
  [S_I_84] -> Subsystem7/5(S5)
  [S_I_85] -> Subsystem7/6(S6)
  qdot_in[9]/1 -> [qdot_in_9]
  S_HVAC[9]/1 -> [S_HVAC_9]
  [BDB_9] -> BDB[9]/1
  [AIB_9] -> AIB[9]/1
  [theta_out_9z] -> theta_out[9]/1
  Subsystem8/1(Sout) -> [S_in_9]
  [S_I_96] -> Subsystem8/7(S7)
  [S_I_97] -> Subsystem8/8(S8)
  [S_I_98] -> Subsystem8/9(S9)
  [S_I_910] -> Subsystem8/10(S10)
  [S_HVAC_9] -> Subsystem8/1(S1)
  [S_I_91] -> Subsystem8/2(S2)
  [S_I_92] -> Subsystem8/3(S3)
  [S_I_93] -> Subsystem8/4(S4)
  [S_I_94] -> Subsystem8/5(S5)
  [S_I_95] -> Subsystem8/6(S6)
  qdot_in[10]/1 -> [qdot_in_10]
  S_HVAC[10]/1 -> [S_HVAC_10]
  [BDB_10] -> BDB[10]/1
  [AIB_10] -> AIB[10]/1
  [theta_out_10z] -> theta_out[10]/1
  Subsystem9/1(Sout) -> [S_in_10]
  [S_I_106] -> Subsystem9/7(S7)
  [S_I_107] -> Subsystem9/8(S8)
  [S_I_108] -> Subsystem9/9(S9)
  [S_I_109] -> Subsystem9/10(S10)
  [S_HVAC_10] -> Subsystem9/1(S1)
  [S_I_101] -> Subsystem9/2(S2)
  [S_I_102] -> Subsystem9/3(S3)
  [S_I_103] -> Subsystem9/4(S4)
  [S_I_104] -> Subsystem9/5(S5)
  [S_I_105] -> Subsystem9/6(S6)
  ZONE_2/1(BDB) -> [BDB_2]
  ZONE_2/2(AIB) -> [AIB_2]
  ZONE_2/3(theta_out) -> [theta_out_2z]
  [qdot_in_2] -> ZONE_2/5(Qdot_in)
  [S_in_2] -> ZONE_2/4(S_in)
  [GDB] -> ZONE_2/2(GDB)
  [WDB] -> ZONE_2/1(WDB)
  [NDB] -> ZONE_2/3(NDB)
  ZONE_3/1(BDB) -> [BDB_3]
  ZONE_3/2(AIB) -> [AIB_3]
  ZONE_3/3(theta_out) -> [theta_out_3z]
  [qdot_in_3] -> ZONE_3/5(Qdot_in)
  [S_in_3] -> ZONE_3/4(S_in)
  [GDB] -> ZONE_3/2(GDB)
  [WDB] -> ZONE_3/1(WDB)
  [NDB] -> ZONE_3/3(NDB)
  ZONE_4/1(BDB) -> [BDB_4]
  ZONE_4/2(AIB) -> [AIB_4]
  ZONE_4/3(theta_out) -> [theta_out_4z]
  [qdot_in_4] -> ZONE_4/5(Qdot_in)
  [S_in_4] -> ZONE_4/4(S_in)
  [GDB] -> ZONE_4/2(GDB)
  [WDB] -> ZONE_4/1(WDB)
  [NDB] -> ZONE_4/3(NDB)
  ZONE_5/1(BDB) -> [BDB_5]
  ZONE_5/2(AIB) -> [AIB_5]
  ZONE_5/3(theta_out) -> [theta_out_5z]
  [qdot_in_5] -> ZONE_5/5(Qdot_in)
  [S_in_5] -> ZONE_5/4(S_in)
  [GDB] -> ZONE_5/2(GDB)
  [WDB] -> ZONE_5/1(WDB)
  [NDB] -> ZONE_5/3(NDB)
  ZONE_6/1(BDB) -> [BDB_6]
  ZONE_6/2(AIB) -> [AIB_6]
  ZONE_6/3(theta_out) -> [theta_out_6z]
  [qdot_in_6] -> ZONE_6/5(Qdot_in)
  [S_in_6] -> ZONE_6/4(S_in)
  [GDB] -> ZONE_6/2(GDB)
  [WDB] -> ZONE_6/1(WDB)
  [NDB] -> ZONE_6/3(NDB)
  ZONE_7/1(BDB) -> [BDB_7]
  ZONE_7/2(AIB) -> [AIB_7]
  ZONE_7/3(theta_out) -> [theta_out_7z]
  [qdot_in_7] -> ZONE_7/5(Qdot_in)
  [S_in_7] -> ZONE_7/4(S_in)
  [GDB] -> ZONE_7/2(GDB)
  [WDB] -> ZONE_7/1(WDB)
  [NDB] -> ZONE_7/3(NDB)
  ZONE_8/1(BDB) -> [BDB_8]
  ZONE_8/2(AIB) -> [AIB_8]
  ZONE_8/3(theta_out) -> [theta_out_8z]
  [qdot_in_8] -> ZONE_8/5(Qdot_in)
  [S_in_8] -> ZONE_8/4(S_in)
  [GDB] -> ZONE_8/2(GDB)
  [WDB] -> ZONE_8/1(WDB)
  [NDB] -> ZONE_8/3(NDB)
  ZONE_9/1(BDB) -> [BDB_9]
  ZONE_9/2(AIB) -> [AIB_9]
  ZONE_9/3(theta_out) -> [theta_out_9z]
  [qdot_in_9] -> ZONE_9/5(Qdot_in)
  [S_in_9] -> ZONE_9/4(S_in)
  [GDB] -> ZONE_9/2(GDB)
  [WDB] -> ZONE_9/1(WDB)
  [NDB] -> ZONE_9/3(NDB)
  ZONE_10/1(BDB) -> [BDB_10]
  ZONE_10/2(AIB) -> [AIB_10]
  ZONE_10/3(theta_out) -> [theta_out_10z]
  [qdot_in_10] -> ZONE_10/5(Qdot_in)
  [S_in_10] -> ZONE_10/4(S_in)
  [GDB] -> ZONE_10/2(GDB)
  [WDB] -> ZONE_10/1(WDB)
  [NDB] -> ZONE_10/3(NDB)
  [control] -> ZONE_1/6(control)
  control/1 -> [control]
  [AIB_1] -> INTERSECTION_1_2/1(AIB1)
  [AIB_2] -> INTERSECTION_1_2/2(AIB2)
  INTERSECTION_1_2/1(S1) -> [S_I_12]
  INTERSECTION_1_2/2(S2) -> [S_I_21]
  [control] -> ZONE_2/6(control)
  [control] -> ZONE_3/6(control)
  [control] -> ZONE_4/6(control)
  [control] -> ZONE_5/6(control)
  [control] -> ZONE_6/6(control)
  [control] -> ZONE_7/6(control)
  [control] -> ZONE_8/6(control)
  [control] -> ZONE_9/6(control)
  [control] -> ZONE_10/6(control)
  [BDB_1] -> INTERSECTION_1_2/3(BDB1)
  [BDB_2] -> INTERSECTION_1_2/4(BDB2)
  [WDB] -> ZONE_1/1(WDB)
  [control] -> INTERSECTION_1_2/5(control)
  [AIB_1] -> INTERSECTION_1_10/1(AIB1)
  [AIB_10] -> INTERSECTION_1_10/2(AIB2)
  INTERSECTION_1_10/1(S1) -> [S_I_110]
  INTERSECTION_1_10/2(S2) -> [S_I_101]
  [BDB_1] -> INTERSECTION_1_10/3(BDB1)
  [BDB_10] -> INTERSECTION_1_10/4(BDB2)
  [control] -> INTERSECTION_1_10/5(control)
  [AIB_1] -> INTERSECTION_1_3/1(AIB1)
  [AIB_3] -> INTERSECTION_1_3/2(AIB2)
  INTERSECTION_1_3/1(S1) -> [S_I_13]
  INTERSECTION_1_3/2(S2) -> [S_I_31]
  [BDB_1] -> INTERSECTION_1_3/3(BDB1)
  [BDB_3] -> INTERSECTION_1_3/4(BDB2)
  [control] -> INTERSECTION_1_3/5(control)
  [AIB_1] -> INTERSECTION_1_4/1(AIB1)
  [AIB_4] -> INTERSECTION_1_4/2(AIB2)
  INTERSECTION_1_4/1(S1) -> [S_I_14]
  INTERSECTION_1_4/2(S2) -> [S_I_41]
  [BDB_1] -> INTERSECTION_1_4/3(BDB1)
  [BDB_4] -> INTERSECTION_1_4/4(BDB2)
  [control] -> INTERSECTION_1_4/5(control)
  [AIB_1] -> INTERSECTION_1_5/1(AIB1)
  [AIB_5] -> INTERSECTION_1_5/2(AIB2)
  INTERSECTION_1_5/1(S1) -> [S_I_15]
  INTERSECTION_1_5/2(S2) -> [S_I_51]
  [BDB_1] -> INTERSECTION_1_5/3(BDB1)
  [BDB_5] -> INTERSECTION_1_5/4(BDB2)
  [control] -> INTERSECTION_1_5/5(control)
  [AIB_1] -> INTERSECTION_1_6/1(AIB1)
  [AIB_6] -> INTERSECTION_1_6/2(AIB2)
  INTERSECTION_1_6/1(S1) -> [S_I_16]
  INTERSECTION_1_6/2(S2) -> [S_I_61]
  [BDB_1] -> INTERSECTION_1_6/3(BDB1)
  [BDB_6] -> INTERSECTION_1_6/4(BDB2)
  [control] -> INTERSECTION_1_6/5(control)
  [AIB_1] -> INTERSECTION_1_7/1(AIB1)
  [AIB_7] -> INTERSECTION_1_7/2(AIB2)
  INTERSECTION_1_7/1(S1) -> [S_I_17]
  INTERSECTION_1_7/2(S2) -> [S_I_71]
  [BDB_1] -> INTERSECTION_1_7/3(BDB1)
  [BDB_7] -> INTERSECTION_1_7/4(BDB2)
  [control] -> INTERSECTION_1_7/5(control)
  [AIB_1] -> INTERSECTION_1_8/1(AIB1)
  [AIB_8] -> INTERSECTION_1_8/2(AIB2)
  INTERSECTION_1_8/1(S1) -> [S_I_18]
  INTERSECTION_1_8/2(S2) -> [S_I_81]
  [BDB_1] -> INTERSECTION_1_8/3(BDB1)
  [BDB_8] -> INTERSECTION_1_8/4(BDB2)
  [control] -> INTERSECTION_1_8/5(control)
  [AIB_1] -> INTERSECTION_1_9/1(AIB1)
  [AIB_9] -> INTERSECTION_1_9/2(AIB2)
  INTERSECTION_1_9/1(S1) -> [S_I_19]
  INTERSECTION_1_9/2(S2) -> [S_I_91]
  [BDB_1] -> INTERSECTION_1_9/3(BDB1)
  [BDB_9] -> INTERSECTION_1_9/4(BDB2)
  [control] -> INTERSECTION_1_9/5(control)
  [AIB_2] -> INTERSECTION_2_3/1(AIB1)
  [AIB_3] -> INTERSECTION_2_3/2(AIB2)
  INTERSECTION_2_3/1(S1) -> [S_I_23]
  INTERSECTION_2_3/2(S2) -> [S_I_32]
  [BDB_2] -> INTERSECTION_2_3/3(BDB1)
  [BDB_3] -> INTERSECTION_2_3/4(BDB2)
  [control] -> INTERSECTION_2_3/5(control)
  [AIB_2] -> INTERSECTION_2_9/1(AIB1)
  [AIB_9] -> INTERSECTION_2_9/2(AIB2)
  INTERSECTION_2_9/1(S1) -> [S_I_29]
  INTERSECTION_2_9/2(S2) -> [S_I_92]
  [BDB_2] -> INTERSECTION_2_9/3(BDB1)
  [BDB_9] -> INTERSECTION_2_9/4(BDB2)
  [control] -> INTERSECTION_2_9/5(control)
  [AIB_2] -> INTERSECTION_2_10/1(AIB1)
  [AIB_10] -> INTERSECTION_2_10/2(AIB2)
  INTERSECTION_2_10/1(S1) -> [S_I_210]
  INTERSECTION_2_10/2(S2) -> [S_I_102]
  [BDB_2] -> INTERSECTION_2_10/3(BDB1)
  [BDB_10] -> INTERSECTION_2_10/4(BDB2)
  [control] -> INTERSECTION_2_10/5(control)
  [AIB_2] -> INTERSECTION_2_4/1(AIB1)
  [AIB_4] -> INTERSECTION_2_4/2(AIB2)
  INTERSECTION_2_4/1(S1) -> [S_I_24]
  INTERSECTION_2_4/2(S2) -> [S_I_42]
  [BDB_2] -> INTERSECTION_2_4/3(BDB1)
  [BDB_4] -> INTERSECTION_2_4/4(BDB2)
  [control] -> INTERSECTION_2_4/5(control)
  [AIB_2] -> INTERSECTION_2_5/1(AIB1)
  [AIB_5] -> INTERSECTION_2_5/2(AIB2)
  INTERSECTION_2_5/1(S1) -> [S_I_25]
  INTERSECTION_2_5/2(S2) -> [S_I_52]
  [BDB_2] -> INTERSECTION_2_5/3(BDB1)
  [BDB_5] -> INTERSECTION_2_5/4(BDB2)
  [control] -> INTERSECTION_2_5/5(control)
  [AIB_2] -> INTERSECTION_2_6/1(AIB1)
  [AIB_6] -> INTERSECTION_2_6/2(AIB2)
  INTERSECTION_2_6/1(S1) -> [S_I_26]
  INTERSECTION_2_6/2(S2) -> [S_I_62]
  [BDB_2] -> INTERSECTION_2_6/3(BDB1)
  [BDB_6] -> INTERSECTION_2_6/4(BDB2)
  [control] -> INTERSECTION_2_6/5(control)
  [AIB_2] -> INTERSECTION_2_7/1(AIB1)
  [AIB_7] -> INTERSECTION_2_7/2(AIB2)
  INTERSECTION_2_7/1(S1) -> [S_I_27]
  INTERSECTION_2_7/2(S2) -> [S_I_72]
  [BDB_2] -> INTERSECTION_2_7/3(BDB1)
  [BDB_7] -> INTERSECTION_2_7/4(BDB2)
  [control] -> INTERSECTION_2_7/5(control)
  [AIB_2] -> INTERSECTION_2_8/1(AIB1)
  [AIB_8] -> INTERSECTION_2_8/2(AIB2)
  INTERSECTION_2_8/1(S1) -> [S_I_28]
  INTERSECTION_2_8/2(S2) -> [S_I_82]
  [BDB_2] -> INTERSECTION_2_8/3(BDB1)
  [BDB_8] -> INTERSECTION_2_8/4(BDB2)
  [control] -> INTERSECTION_2_8/5(control)
  [AIB_3] -> INTERSECTION_3_4/1(AIB1)
  [AIB_4] -> INTERSECTION_3_4/2(AIB2)
  INTERSECTION_3_4/1(S1) -> [S_I_34]
  INTERSECTION_3_4/2(S2) -> [S_I_43]
  [BDB_3] -> INTERSECTION_3_4/3(BDB1)
  [BDB_4] -> INTERSECTION_3_4/4(BDB2)
  [control] -> INTERSECTION_3_4/5(control)
  [AIB_3] -> INTERSECTION_3_5/1(AIB1)
  [AIB_5] -> INTERSECTION_3_5/2(AIB2)
  INTERSECTION_3_5/1(S1) -> [S_I_35]
  INTERSECTION_3_5/2(S2) -> [S_I_53]
  [BDB_3] -> INTERSECTION_3_5/3(BDB1)
  [BDB_5] -> INTERSECTION_3_5/4(BDB2)
  [control] -> INTERSECTION_3_5/5(control)
  [AIB_3] -> INTERSECTION_3_6/1(AIB1)
  [AIB_6] -> INTERSECTION_3_6/2(AIB2)
  INTERSECTION_3_6/1(S1) -> [S_I_36]
  INTERSECTION_3_6/2(S2) -> [S_I_63]
  [BDB_3] -> INTERSECTION_3_6/3(BDB1)
  [BDB_6] -> INTERSECTION_3_6/4(BDB2)
  [control] -> INTERSECTION_3_6/5(control)
  [AIB_3] -> INTERSECTION_3_7/1(AIB1)
  [AIB_7] -> INTERSECTION_3_7/2(AIB2)
  INTERSECTION_3_7/1(S1) -> [S_I_37]
  INTERSECTION_3_7/2(S2) -> [S_I_73]
  [BDB_3] -> INTERSECTION_3_7/3(BDB1)
  [BDB_7] -> INTERSECTION_3_7/4(BDB2)
  [control] -> INTERSECTION_3_7/5(control)
  [AIB_3] -> INTERSECTION_3_8/1(AIB1)
  [AIB_8] -> INTERSECTION_3_8/2(AIB2)
  INTERSECTION_3_8/1(S1) -> [S_I_38]
  INTERSECTION_3_8/2(S2) -> [S_I_83]
  [BDB_3] -> INTERSECTION_3_8/3(BDB1)
  [BDB_8] -> INTERSECTION_3_8/4(BDB2)
  [control] -> INTERSECTION_3_8/5(control)
  [AIB_3] -> INTERSECTION_3_9/1(AIB1)
  [AIB_9] -> INTERSECTION_3_9/2(AIB2)
  INTERSECTION_3_9/1(S1) -> [S_I_39]
  INTERSECTION_3_9/2(S2) -> [S_I_93]
  [BDB_3] -> INTERSECTION_3_9/3(BDB1)
  [BDB_9] -> INTERSECTION_3_9/4(BDB2)
  [control] -> INTERSECTION_3_9/5(control)
  [AIB_3] -> INTERSECTION_3_10/1(AIB1)
  [AIB_10] -> INTERSECTION_3_10/2(AIB2)
  INTERSECTION_3_10/1(S1) -> [S_I_310]
  INTERSECTION_3_10/2(S2) -> [S_I_103]
  [BDB_3] -> INTERSECTION_3_10/3(BDB1)
  [BDB_10] -> INTERSECTION_3_10/4(BDB2)
  [control] -> INTERSECTION_3_10/5(control)
  [AIB_4] -> INTERSECTION_4_5/1(AIB1)
  [AIB_5] -> INTERSECTION_4_5/2(AIB2)
  INTERSECTION_4_5/1(S1) -> [S_I_45]
  INTERSECTION_4_5/2(S2) -> [S_I_54]
  [BDB_4] -> INTERSECTION_4_5/3(BDB1)
  [BDB_5] -> INTERSECTION_4_5/4(BDB2)
  [control] -> INTERSECTION_4_5/5(control)
  [AIB_4] -> INTERSECTION_4_6/1(AIB1)
  [AIB_6] -> INTERSECTION_4_6/2(AIB2)
  INTERSECTION_4_6/1(S1) -> [S_I_46]
  INTERSECTION_4_6/2(S2) -> [S_I_64]
  [BDB_4] -> INTERSECTION_4_6/3(BDB1)
  [BDB_6] -> INTERSECTION_4_6/4(BDB2)
  [control] -> INTERSECTION_4_6/5(control)
  [AIB_4] -> INTERSECTION_4_7/1(AIB1)
  [AIB_7] -> INTERSECTION_4_7/2(AIB2)
  INTERSECTION_4_7/1(S1) -> [S_I_47]
  INTERSECTION_4_7/2(S2) -> [S_I_74]
  [BDB_4] -> INTERSECTION_4_7/3(BDB1)
  [BDB_7] -> INTERSECTION_4_7/4(BDB2)
  [control] -> INTERSECTION_4_7/5(control)
  [AIB_4] -> INTERSECTION_4_8/1(AIB1)
  [AIB_8] -> INTERSECTION_4_8/2(AIB2)
  INTERSECTION_4_8/1(S1) -> [S_I_48]
  INTERSECTION_4_8/2(S2) -> [S_I_84]
  [BDB_4] -> INTERSECTION_4_8/3(BDB1)
  [BDB_8] -> INTERSECTION_4_8/4(BDB2)
  [control] -> INTERSECTION_4_8/5(control)
  [AIB_4] -> INTERSECTION_4_9/1(AIB1)
  [AIB_9] -> INTERSECTION_4_9/2(AIB2)
  INTERSECTION_4_9/1(S1) -> [S_I_49]
  INTERSECTION_4_9/2(S2) -> [S_I_94]
  [BDB_4] -> INTERSECTION_4_9/3(BDB1)
  [BDB_9] -> INTERSECTION_4_9/4(BDB2)
  [control] -> INTERSECTION_4_9/5(control)
  [AIB_4] -> INTERSECTION_4_10/1(AIB1)
  [AIB_10] -> INTERSECTION_4_10/2(AIB2)
  INTERSECTION_4_10/1(S1) -> [S_I_410]
  INTERSECTION_4_10/2(S2) -> [S_I_104]
  [BDB_4] -> INTERSECTION_4_10/3(BDB1)
  [BDB_10] -> INTERSECTION_4_10/4(BDB2)
  [control] -> INTERSECTION_4_10/5(control)
  [AIB_5] -> INTERSECTION_5_6/1(AIB1)
  [AIB_6] -> INTERSECTION_5_6/2(AIB2)
  INTERSECTION_5_6/1(S1) -> [S_I_56]
  INTERSECTION_5_6/2(S2) -> [S_I_65]
  [BDB_5] -> INTERSECTION_5_6/3(BDB1)
  [BDB_6] -> INTERSECTION_5_6/4(BDB2)
  [control] -> INTERSECTION_5_6/5(control)
  [AIB_5] -> INTERSECTION_5_7/1(AIB1)
  [AIB_7] -> INTERSECTION_5_7/2(AIB2)
  INTERSECTION_5_7/1(S1) -> [S_I_57]
  INTERSECTION_5_7/2(S2) -> [S_I_75]
  [BDB_5] -> INTERSECTION_5_7/3(BDB1)
  [BDB_7] -> INTERSECTION_5_7/4(BDB2)
  [control] -> INTERSECTION_5_7/5(control)
  [AIB_5] -> INTERSECTION_5_8/1(AIB1)
  [AIB_8] -> INTERSECTION_5_8/2(AIB2)
  INTERSECTION_5_8/1(S1) -> [S_I_58]
  INTERSECTION_5_8/2(S2) -> [S_I_85]
  [BDB_5] -> INTERSECTION_5_8/3(BDB1)
  [BDB_8] -> INTERSECTION_5_8/4(BDB2)
  [control] -> INTERSECTION_5_8/5(control)
  [AIB_5] -> INTERSECTION_5_9/1(AIB1)
  [AIB_9] -> INTERSECTION_5_9/2(AIB2)
  INTERSECTION_5_9/1(S1) -> [S_I_59]
  INTERSECTION_5_9/2(S2) -> [S_I_95]
  [BDB_5] -> INTERSECTION_5_9/3(BDB1)
  [BDB_9] -> INTERSECTION_5_9/4(BDB2)
  [control] -> INTERSECTION_5_9/5(control)
  [AIB_5] -> INTERSECTION_5_10/1(AIB1)
  [AIB_10] -> INTERSECTION_5_10/2(AIB2)
  INTERSECTION_5_10/1(S1) -> [S_I_510]
  INTERSECTION_5_10/2(S2) -> [S_I_105]
  [BDB_5] -> INTERSECTION_5_10/3(BDB1)
  [BDB_10] -> INTERSECTION_5_10/4(BDB2)
  [control] -> INTERSECTION_5_10/5(control)
  [AIB_6] -> INTERSECTION_6_7/1(AIB1)
  [AIB_7] -> INTERSECTION_6_7/2(AIB2)
  INTERSECTION_6_7/1(S1) -> [S_I_67]
  INTERSECTION_6_7/2(S2) -> [S_I_76]
  [BDB_6] -> INTERSECTION_6_7/3(BDB1)
  [BDB_7] -> INTERSECTION_6_7/4(BDB2)
  [control] -> INTERSECTION_6_7/5(control)
  [AIB_6] -> INTERSECTION_6_8/1(AIB1)
  [AIB_8] -> INTERSECTION_6_8/2(AIB2)
  INTERSECTION_6_8/1(S1) -> [S_I_68]
  INTERSECTION_6_8/2(S2) -> [S_I_86]
  [BDB_6] -> INTERSECTION_6_8/3(BDB1)
  [BDB_8] -> INTERSECTION_6_8/4(BDB2)
  [control] -> INTERSECTION_6_8/5(control)
  [AIB_6] -> INTERSECTION_6_9/1(AIB1)
  [AIB_9] -> INTERSECTION_6_9/2(AIB2)
  INTERSECTION_6_9/1(S1) -> [S_I_69]
  INTERSECTION_6_9/2(S2) -> [S_I_96]
  [BDB_6] -> INTERSECTION_6_9/3(BDB1)
  [BDB_9] -> INTERSECTION_6_9/4(BDB2)
  [control] -> INTERSECTION_6_9/5(control)
  [AIB_6] -> INTERSECTION_6_10/1(AIB1)
  [AIB_10] -> INTERSECTION_6_10/2(AIB2)
  INTERSECTION_6_10/1(S1) -> [S_I_610]
  INTERSECTION_6_10/2(S2) -> [S_I_106]
  [BDB_6] -> INTERSECTION_6_10/3(BDB1)
  [BDB_10] -> INTERSECTION_6_10/4(BDB2)
  [control] -> INTERSECTION_6_10/5(control)
  [AIB_7] -> INTERSECTION_7_8/1(AIB1)
  [AIB_8] -> INTERSECTION_7_8/2(AIB2)
  INTERSECTION_7_8/1(S1) -> [S_I_78]
  INTERSECTION_7_8/2(S2) -> [S_I_87]
  [BDB_7] -> INTERSECTION_7_8/3(BDB1)
  [BDB_8] -> INTERSECTION_7_8/4(BDB2)
  [control] -> INTERSECTION_7_8/5(control)
  [AIB_7] -> INTERSECTION_7_9/1(AIB1)
  [AIB_9] -> INTERSECTION_7_9/2(AIB2)
  INTERSECTION_7_9/1(S1) -> [S_I_79]
  INTERSECTION_7_9/2(S2) -> [S_I_97]
  [BDB_7] -> INTERSECTION_7_9/3(BDB1)
  [BDB_9] -> INTERSECTION_7_9/4(BDB2)
  [control] -> INTERSECTION_7_9/5(control)
  [AIB_7] -> INTERSECTION_7_10/1(AIB1)
  [AIB_10] -> INTERSECTION_7_10/2(AIB2)
  INTERSECTION_7_10/1(S1) -> [S_I_710]
  INTERSECTION_7_10/2(S2) -> [S_I_107]
  [BDB_7] -> INTERSECTION_7_10/3(BDB1)
  [BDB_10] -> INTERSECTION_7_10/4(BDB2)
  [control] -> INTERSECTION_7_10/5(control)
  [AIB_8] -> INTERSECTION_8_9/1(AIB1)
  [AIB_9] -> INTERSECTION_8_9/2(AIB2)
  INTERSECTION_8_9/1(S1) -> [S_I_89]
  INTERSECTION_8_9/2(S2) -> [S_I_98]
  [BDB_8] -> INTERSECTION_8_9/3(BDB1)
  [BDB_9] -> INTERSECTION_8_9/4(BDB2)
  [control] -> INTERSECTION_8_9/5(control)
  [AIB_8] -> INTERSECTION_8_10/1(AIB1)
  [AIB_10] -> INTERSECTION_8_10/2(AIB2)
  INTERSECTION_8_10/1(S1) -> [S_I_810]
  INTERSECTION_8_10/2(S2) -> [S_I_108]
  [BDB_8] -> INTERSECTION_8_10/3(BDB1)
  [BDB_10] -> INTERSECTION_8_10/4(BDB2)
  [control] -> INTERSECTION_8_10/5(control)
  [AIB_9] -> INTERSECTION_9_10/1(AIB1)
  [AIB_10] -> INTERSECTION_9_10/2(AIB2)
  INTERSECTION_9_10/1(S1) -> [S_I_910]
  INTERSECTION_9_10/2(S2) -> [S_I_109]
  [BDB_9] -> INTERSECTION_9_10/3(BDB1)
  [BDB_10] -> INTERSECTION_9_10/4(BDB2)
  [control] -> INTERSECTION_9_10/5(control)
